simulink model "Control_Telegram"  (R2020b)
settings: Solver=FixedStepDiscrete  StartTime=0.0  StopTime=inf  FixedStep=0.01  RelTol=1e-3  EnableMultiTasking=on
libraries: arduinolib x12, simulink x4, pid_lib x2, commutil2 x1
settings Model: SILPILModeSetting=veronly  ExtModeTrigDuration=2  Creator=Lenovo  LastModifiedBy=Lenovo
settings SolverCC: AutoInsertRateTranBlk=on
settings OptimizationCC: EnhancedBackFolding=on  PassReuseOutputArgsAs=Individual arguments  ZeroExternalMemoryAtStartup=off  ZeroInternalMemoryAtStartup=off  MaxStackSize=64  OptimizeBlockOrder=speed  DifferentSizesBufferReuse=on  OptimizationCustomize=off  EfficientTunableParamExpr=on
settings DebuggingCC: MultiTaskDSMMsg=none  ParameterTunabilityLossMsg=error
settings HardwareCC: ProdBitPerInt=16  ProdBitPerPointer=16  ProdBitPerSizeT=16  ProdBitPerPtrDiffT=16  ProdLargestAtomicFloat=None  ProdWordSize=8  ProdHWDeviceType=Atmel->AVR
settings SFSimCC: MATLABDynamicMemAlloc=off
settings RTWCC: Description=Embedded Coder  SystemTargetFile=ert.tlc  HardwareBoard=Arduino Mega 2560  TemplateMakefile=ert_default_tmf  Toolchain=Arduino AVR  BuildConfiguration=Faster Runs
settings CodeAppCC: ForceParamTrailComments=on  IgnoreCustomStorageClasses=off  OperatorAnnotations=on  SimulinkDataObjDesc=on  SFDataObjDesc=on  InsertBlockDesc=on
settings ERTTargetCC: SupportContinuousTime=on  SupportVariableSizeSignals=on  ExtModeStaticAllocSize=2048

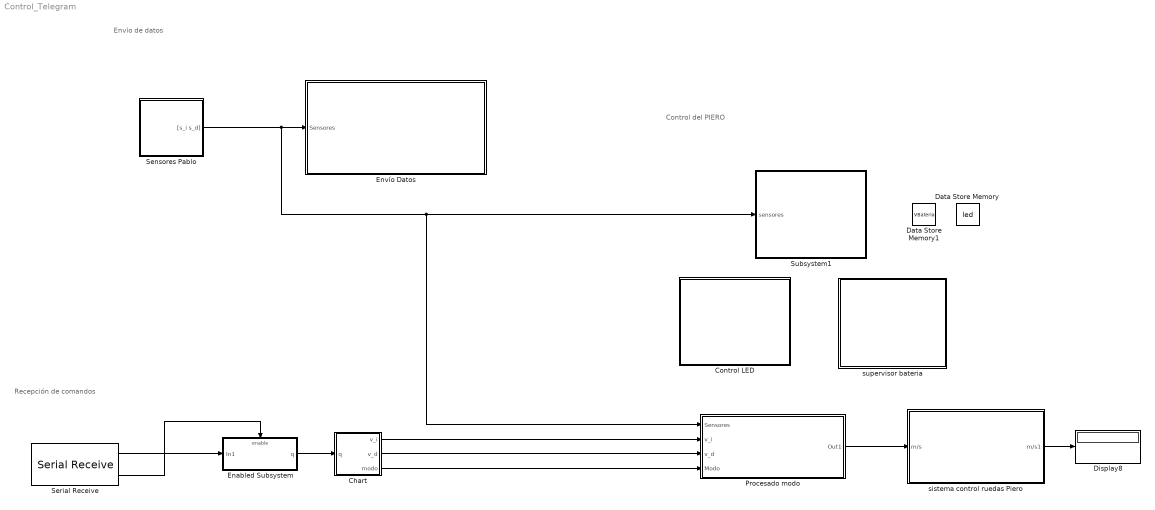
== system Control_Telegram ==
  note: Recepción de comandos
  note: Control del PIERO
  note: Envío de datos
  Chart : Stateflow chart  TreatAsAtomicUnit=on
      settings: PortSchema="{\"entries\":[{\"content\":{\"sides\":[{\"content\":{\"connectorIds\":[\"In1\"]},\"type\":\"ConnectorPlacement.EquallySpacedRectSide\",\"uuid\":\"460ffd16-b0a8-46f0-b413-d255944a2202\"},{\"content\":{\"connectorIds\":[\"Out2\",\"Out1\",\"Out3\"],\"side\":\"RIGHT\"},\"type\":\"ConnectorPlacement.EquallySpacedRectSide\",\"uuid\":\"2f6da82c-ccd3-4a6a-9034-5a862735bd5f\"},{\"content\":{\"connectorIds\":[],\"side\":\"TOP\"},\"type\":\"ConnectorPlacement.EquallySpacedRectSide\",\"uuid\":\"193d4201-0e4c-4dc7-8b4f-a6b3a7c4f850\"},{\"content\":{\"connectorIds\":[],\"side\":\"HIDDEN\"},\"type\":\"ConnectorPlacement.EquallySpacedRectSide\",\"uuid\":\"5c8087d8-0ec6-4d7b-ac7b-a5b39b248132\"}]},\"type\":\"ConnectorPlacement.EquallySpacedConnector\",\"uuid\":\"9f9eacda-d61e-4b8a-833c-1ceadcf75f15\"}],\"packageUris\":[\"http://schema.mathworks.com/mf0/Connector/R2020b\"],\"version\":\"1.0\"}"
  Control LED : Subsystem
      mask Display: image('C:\Users\Lenovo\Desktop\4ºGIERM\LAB ROB\RBG-LED.jpg'); % Use "Edit Image" on toolstrip to change.
  Data Store Memory : DataStoreMemory  DataStoreName=led  ReadBeforeWriteMsg=warning  WriteAfterWriteMsg=warning  WriteAfterReadMsg=warning  ShowAdditionalParam=off
  Data Store Memory1 : DataStoreMemory  DataStoreName=VBateria  ReadBeforeWriteMsg=warning  WriteAfterWriteMsg=warning  WriteAfterReadMsg=warning  ShowAdditionalParam=off
  Display8 : Display
  Enabled Subsystem : Subsystem  TreatAsAtomicUnit=on
  Envío Datos : Subsystem
  Procesado modo : Subsystem
  Sensores Pablo : Subsystem
      mask Display: image('C:\Users\Lenovo\Desktop\4ºGIERM\LAB ROB\sensor.jpg'); % Use "Edit Image" on toolstrip to change.
  Serial Receive : arduinolib/Serial Receive  isARMArch=off  portNumber=3  DataType=uint8  Datalength=1  SampleTime=0.01  showOutStatus=on  blockPlatform=arduino
      settings: SourceProductBaseCode=ARDUINO
  Subsystem1 : Subsystem
  sistema control ruedas Piero : Subsystem
  supervisor bateria : Subsystem
      mask Display: image('C:\Users\Lenovo\Desktop\4ºGIERM\LAB ROB\bateria.jpg'); % Use "Edit Image" on toolstrip to change.
  wires:
  Serial Receive/2 -> Enabled Subsystem/Enable
  Sensores Pablo/1("[s_i s_d]") -> Procesado modo/1(Sensores), Subsystem1/1(sensores), Envío Datos/1(Sensores)
  Enabled Subsystem/1(q) -> Chart/1(q)
  Serial Receive/1 -> Enabled Subsystem/1(In1)
  sistema control ruedas Piero/1(m/s1) -> Display8/1
  Chart/2(v_i) -> Procesado modo/2(v_i)
  Chart/1(v_d) -> Procesado modo/3(v_d)
  Chart/3(modo) -> Procesado modo/4(Modo)
  Procesado modo/1(Out1) -> sistema control ruedas Piero/1(m/s)

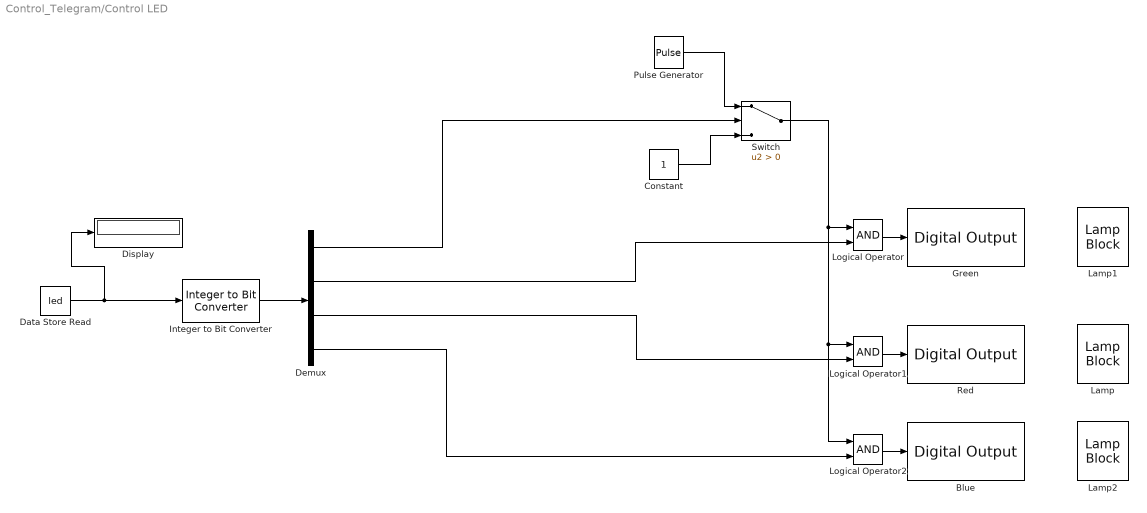
== system Control_Telegram/Control LED ==
  Blue : arduinolib/Digital Output  pinNumber=49  Direction=output  blockPlatform=arduino
  Constant : Constant
  Data Store Read : DataStoreRead  DataStoreName=led
  Demux : Demux
  Display : Display
  Green : arduinolib/Digital Output  pinNumber=53  Direction=output  blockPlatform=arduino
  Integer to Bit Converter : commutil2/Integer to Bit Converter  nbits=4  signedInputValues=Unsigned  bitOrder=MSB first  outDtype=Inherit via internal rule
  Lamp : LampBlock
  Lamp1 : LampBlock
  Lamp2 : LampBlock
  Logical Operator : Logic  AllPortsSameDT=off  OutDataTypeStr=boolean
  Logical Operator1 : Logic  AllPortsSameDT=off  OutDataTypeStr=boolean
  Logical Operator2 : Logic  AllPortsSameDT=off  OutDataTypeStr=boolean
  Pulse Generator : DiscretePulseGenerator  PulseType=Time based  Period=0.5  PulseWidth=50
  Red : arduinolib/Digital Output  pinNumber=51  Direction=output  blockPlatform=arduino
  Switch : Switch  Criteria=u2 > Threshold
  wires:
  Logical Operator/1 -> Green/1
  Logical Operator2/1 -> Blue/1
  Logical Operator1/1 -> Red/1
  Switch/1 -> Logical Operator2/1, Logical Operator1/1, Logical Operator/1
  Demux/1 -> Switch/2
  Pulse Generator/1 -> Switch/1
  Constant/1 -> Switch/3
  Data Store Read/1 -> Display/1, Integer to Bit Converter/1
  Demux/2 -> Logical Operator/2
  Demux/4 -> Logical Operator2/2
  Demux/3 -> Logical Operator1/2
  Integer to Bit Converter/1 -> Demux/1

== system Control_Telegram/Enabled Subsystem ==
  In1 : Inport
  Enable : EnablePort
  q : Outport
  wires:
  In1/1 -> q/1

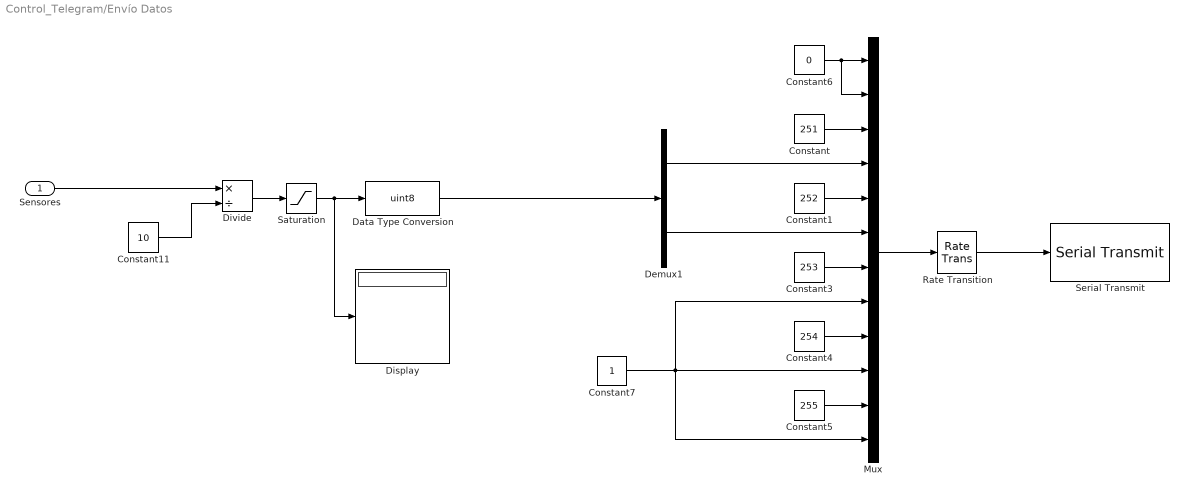
== system Control_Telegram/Envío Datos ==
  Sensores : Inport
  Constant : Constant  Value=251  OutDataTypeStr=uint8
  Constant1 : Constant  Value=252  OutDataTypeStr=uint8
  Constant11 : Constant  Value=10
  Constant3 : Constant  Value=253  OutDataTypeStr=uint8
  Constant4 : Constant  Value=254  OutDataTypeStr=uint8
  Constant5 : Constant  Value=255  OutDataTypeStr=uint8
  Constant6 : Constant  Value=0  OutDataTypeStr=uint8
  Constant7 : Constant  OutDataTypeStr=uint8
  Data Type Conversion : DataTypeConversion  OutMax=250  OutDataTypeStr=uint8
  Demux1 : Demux  Outputs=2
  Display : Display
  Divide : Product  Inputs=*/
  Mux : Mux  Inputs=12
  Rate Transition : RateTransition  OutPortSampleTime=0.9
  Saturation : Saturate  UpperLimit=255  LowerLimit=0
  Serial Transmit : arduinolib/Serial Transmit  portNumber=3  sendmode=write  label=sensores  sendformat=Decimal  floatprecision=2  blockPlatform=arduino
  wires:
  Constant5/1 -> Mux/11
  Rate Transition/1 -> Serial Transmit/1
  Constant3/1 -> Mux/7
  Constant6/1 -> Mux/2, Mux/1
  Saturation/1 -> Display/1, Data Type Conversion/1
  Demux1/1 -> Mux/4
  Constant4/1 -> Mux/9
  Mux/1 -> Rate Transition/1
  Constant1/1 -> Mux/5
  Divide/1 -> Saturation/1
  Data Type Conversion/1 -> Demux1/1
  Constant7/1 -> Mux/12, Mux/10, Mux/8
  Demux1/2 -> Mux/6
  Constant11/1 -> Divide/2
  Constant/1 -> Mux/3
  Sensores/1 -> Divide/1

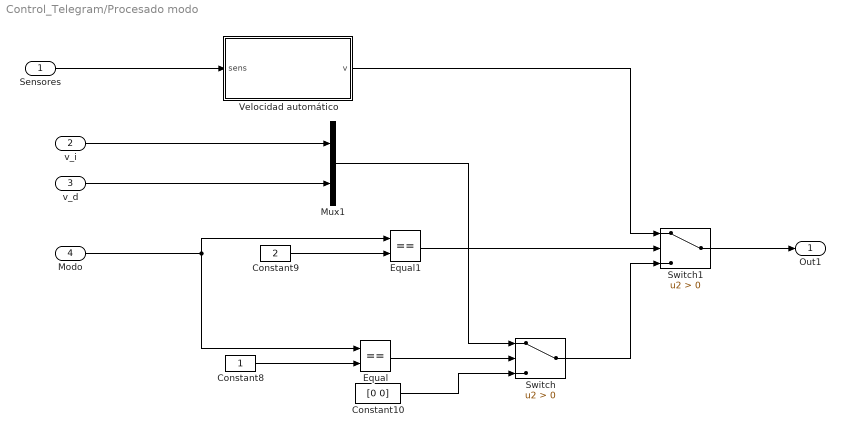
== system Control_Telegram/Procesado modo ==
  Sensores : Inport
  v_i : Inport  Port=2
  v_d : Inport  Port=3
  Modo : Inport  Port=4
  Constant10 : Constant  Value=[0 0]
  Constant8 : Constant
  Constant9 : Constant  Value=2
  Equal : RelationalOperator  Operator===  OutDataTypeStr=boolean  RndMeth=Simplest
  Equal1 : RelationalOperator  Operator===  OutDataTypeStr=boolean  RndMeth=Simplest
  Mux1 : Mux  Inputs=2
  Switch : Switch  Criteria=u2 > Threshold
  Switch1 : Switch  Criteria=u2 > Threshold
  Velocidad automático : Subsystem
  Out1 : Outport
  wires:
  Equal1/1 -> Switch1/2
  Equal/1 -> Switch/2
  Modo/1 -> Equal1/1, Equal/1
  Mux1/1 -> Switch/1
  Switch/1 -> Switch1/3
  v_d/1 -> Mux1/2
  Switch1/1 -> Out1/1
  Constant8/1 -> Equal/2
  Constant10/1 -> Switch/3
  Constant9/1 -> Equal1/2
  v_i/1 -> Mux1/1
  Sensores/1 -> Velocidad automático/1(sens)
  Velocidad automático/1(v) -> Switch1/1

== system Control_Telegram/Sensores Pablo ==
  Display2 : Display
  Display3 : Display
  Mux : Mux  Inputs=2
  SENSORES : Subsystem
  "[s_i s_d]" : Outport
  wires:
  SENSORES/2(Sensor Derecho) -> Mux/2, Display3/1
  SENSORES/1(Sensor Izquierdo) -> Mux/1, Display2/1
  Mux/1 -> "[s_i s_d]"/1

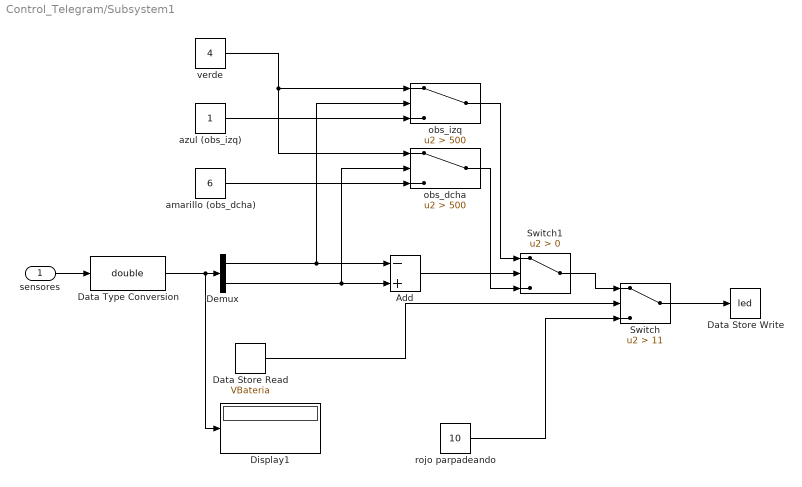
== system Control_Telegram/Subsystem1 ==
  sensores : Inport
  Add : Sum  Inputs=-+
  Data Store Read : DataStoreRead  DataStoreName=VBateria
  Data Store Write : DataStoreWrite  DataStoreName=led
  Data Type Conversion : DataTypeConversion  OutDataTypeStr=double
  Demux : Demux  Outputs=2
  Display1 : Display
  Switch : Switch  Criteria=u2 > Threshold  Threshold=11
  Switch1 : Switch  Criteria=u2 > Threshold
  amarillo (obs_dcha) : Constant  Value=6
  azul (obs_izq) : Constant
  obs_dcha : Switch  Criteria=u2 > Threshold  Threshold=500
  obs_izq : Switch  Criteria=u2 > Threshold  Threshold=500
  rojo parpadeando : Constant  Value=10
  verde : Constant  Value=4
  wires:
  Switch/1 -> Data Store Write/1
  rojo parpadeando/1 -> Switch/3
  sensores/1 -> Data Type Conversion/1
  verde/1 -> obs_izq/1, obs_dcha/1
  Demux/1 -> Add/1, obs_izq/2
  Demux/2 -> Add/2, obs_dcha/2
  azul (obs_izq)/1 -> obs_izq/3
  amarillo (obs_dcha)/1 -> obs_dcha/3
  Switch1/1 -> Switch/1
  Add/1 -> Switch1/2
  obs_izq/1 -> Switch1/1
  obs_dcha/1 -> Switch1/3
  Data Store Read/1 -> Switch/2
  Data Type Conversion/1 -> Display1/1, Demux/1

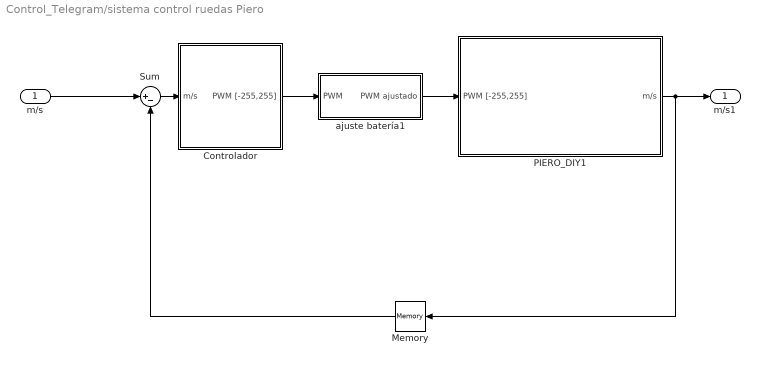
== system Control_Telegram/sistema control ruedas Piero ==
  m/s : Inport
  Controlador : Subsystem
  Memory : Memory
  PIERO_DIY1 : Subsystem
  Sum : Sum  Inputs=|+-
  ajuste batería1 : Subsystem
  m/s1 : Outport  VectorParamsAs1DForOutWhenUnconnected=off
  wires:
  Sum/1 -> Controlador/1(m/s)
  m/s/1 -> Sum/1
  PIERO_DIY1/1(m/s) -> Memory/1, m/s1/1
  Memory/1 -> Sum/2
  Controlador/1(PWM [-255,255]) -> ajuste batería1/1(PWM)
  ajuste batería1/1(PWM ajustado) -> PIERO_DIY1/1(PWM [-255,255])

== system Control_Telegram/supervisor bateria ==
  Bateria : arduinolib/Analog Input  pinNumber=0  ReadResultsOnly=off  ConversionTriggerSource=Software  ExternalTriggerType=uint32( 0 )  OutputDataType=uint16  EnableConversionCompleteNotify=off  EnableOuputStatus=off  SampleTime=1  blockPlatform=arduino
  Data Store Write1 : DataStoreWrite  DataStoreName=VBateria
  Gain : Gain  Gain=25/1023  OutDataTypeStr=double
  Quarter Gauge : QuarterGaugeBlock  ScaleMin=10  ScaleMax=13
  wires:
  Bateria/1 -> Gain/1
  Gain/1 -> Data Store Write1/1

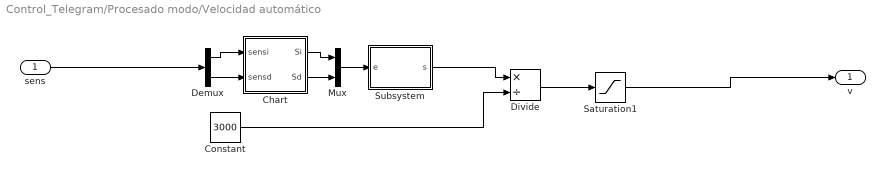
== system Control_Telegram/Procesado modo/Velocidad automático ==
  sens : Inport
  Chart : Stateflow chart  TreatAsAtomicUnit=on
  Constant : Constant  Value=3000
  Demux : Demux  Outputs=2
  Divide : Product  Inputs=*/
  Mux : Mux  Inputs=2
  Saturation1 : Saturate  UpperLimit=0.3  LowerLimit=0
  Subsystem : Subsystem
      settings: PortSchema="{\"entries\":[{\"content\":{\"sides\":[{\"content\":{\"connectorIds\":[]},\"type\":\"ConnectorPlacement.EquallySpacedRectSide\",\"uuid\":\"0a24279a-7a52-457c-98aa-c7ba1e82fcaa\"},{\"content\":{\"connectorIds\":[],\"side\":\"RIGHT\"},\"type\":\"ConnectorPlacement.EquallySpacedRectSide\",\"uuid\":\"0f762eb3-cf5d-4914-a9fc-c3582c9f6173\"},{\"content\":{\"connectorIds\":[\"In1\"],\"side\":\"TOP\"},\"type\":\"ConnectorPlacement.EquallySpacedRectSide\",\"uuid\":\"ea3e191d-7b8c-4d85-afaf-b1ec388f1efb\"},{\"content\":{\"connectorIds\":[\"Out1\"],\"side\":\"BOTTOM\"},\"type\":\"ConnectorPlacement.EquallySpacedRectSide\",\"uuid\":\"8d5bc53a-83b0-4fc8-aeef-cd0991329a34\"},{\"content\":{\"connectorIds\":[],\"side\":\"HIDDEN\"},\"type\":\"ConnectorPlacement.EquallySpacedRectSide\",\"uuid\":\"6d880959-49a3-460c-8ffc-802dbf3ca6c3\"}]},\"type\":\"ConnectorPlacement.EquallySpacedConnector\",\"uuid\":\"f1470ebd-e65e-4dba-8453-0009f24bd770\"}],\"packageUris\":[\"http://schema.mathworks.com/mf0/Connector/R2020b\"],\"version\":\"1.0\"}"
  v : Outport
  wires:
  Divide/1 -> Saturation1/1
  Saturation1/1 -> v/1
  Constant/1 -> Divide/2
  sens/1 -> Demux/1
  Demux/1 -> Chart/1(sensi)
  Chart/1(Si) -> Mux/1
  Demux/2 -> Chart/2(sensd)
  Chart/2(Sd) -> Mux/2
  Mux/1 -> Subsystem/1(e)
  Subsystem/1(s) -> Divide/1

== system Control_Telegram/Sensores Pablo/SENSORES ==
  Display : Display
  Display1 : Display
  S-Function Builder : S-Function  InitFcn=try, set_param(gcb,'FunctionName','Sensores_VL53L0X_I2C'), end  FunctionName=Sensores_VL53L0X_I2C  SFunctionModules=Sensores_VL53L0X_I2C_wrapper  SFunctionDeploymentMode=off  EnableBusSupport=off  mask(S-Function Builder){}
      mask help: Simulink:masks:SFunctionBuilder_MD
      mask init:
      | val = [[.9  0.75 0.75 1 1 .9 .9 1]',[1 1 0.75 0.75 .9 .9 1 .9]'];try , sys = get_param(gcb,'SfunBuilderFcnName');if isempty(sys), sys = get_param(gcb,'FunctionName'); end,catch, sys = get_param(gcb,'FunctionName'); end
      settings: CopyFcn=set_param(gcbh,'LinkStatus','none')  PreSaveFcn=try, set_param(gcb,'FunctionName','Sensores_VL53L0X_I2C'), end  OpenFcn=sfunctionwizard(gcbh)
      mask Display: plot(val(:,1),val(:,2)),disp(sys),port_label('output',1,'Sensor1'),port_label('output',2,'Sensor2')
  Sensor Izquierdo : Outport  VectorParamsAs1DForOutWhenUnconnected=off
  Sensor Derecho : Outport  Port=2  VectorParamsAs1DForOutWhenUnconnected=off
  wires:
  S-Function Builder/2 -> Display/1, Sensor Derecho/1
  S-Function Builder/1 -> Display1/1, Sensor Izquierdo/1

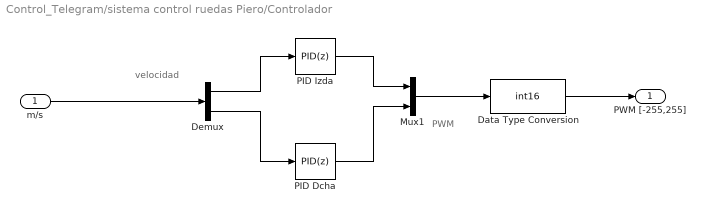
== system Control_Telegram/sistema control ruedas Piero/Controlador ==
  note: velocidad
  note: PWM
  m/s : Inport
  Data Type Conversion : DataTypeConversion  OutDataTypeStr=int16
  Demux : Demux  Outputs=2
  Mux1 : Mux  Inputs=2
  PID Dcha : pid_lib/PID Controller  Controller=PID  Form=Parallel  TimeDomain=Discrete-time  UseExternalTs=off  SampleTime=-1  IntegratorMethod=Forward Euler  FilterMethod=Forward Euler  ControllerParametersSource=internal  P=4.07505423535344  I=815.010847070688  D=0  UseFilter=on  N=100  TunerSelectOption=Transfer Function Based (PID Tuner App)  InitialConditionSource=internal  InitialConditionForIntegrator=0  InitialConditionForFilter=0  DifferentiatorICPrevScaledInput=0  ExternalReset=none  TrackingMode=off  Kt=1  LimitOutput=on  SatLimitsSource=internal  UpperSaturationLimit=255  LowerSaturationLimit=-255  LinearizeAsGain=on  AntiWindupMode=none  Kb=1  POutMin=[]  POutMax=[]  IOutMin=[]  IOutMax=[]  DOutMin=[]  DOutMax=[]  NOutMin=[]  NOutMax=[]  SumOutMin=[]  SumOutMax=[]  SaturationOutMin=[]  SaturationOutMax=[]  PParamMin=[]  PParamMax=[]  IParamMin=[]  IParamMax=[]  DParamMin=[]  DParamMax=[]  NParamMin=[]  NParamMax=[]  KbParamMin=[]  KbParamMax=[]  KtParamMin=[]  KtParamMax=[]  KbOutMin=[]  KbOutMax=[]  KtOutMin=[]  KtOutMax=[]  IntegratorOutMin=[]  IntegratorOutMax=[]  FilterOutMin=[]  FilterOutMax=[]  SumI1OutMin=[]  SumI1OutMax=[]  SumI2OutMin=[]  SumI2OutMax=[]  SumI3OutMin=[]  SumI3OutMax=[]  SumI4OutMin=[]  SumI4OutMax=[]  SumDOutMin=[]  SumDOutMax=[]  DifferentiatorOutMin=[]  DifferentiatorOutMax=[]  FilterDiffOutCoefMin=[]  FilterDiffOutCoefMax=[]  ReciprocalOutMin=[]  ReciprocalOutMax=[]  SumDenOutMin=[]  SumDenOutMax=[]  SumNumOutMin=[]  SumNumOutMax=[]  DivideOutMin=[]  DivideOutMax=[]  UdiffTsProdOutMin=[]  UdiffTsProdOutMax=[]  NTsProdOutMin=[]  NTsProdOutMax=[]  UintegralTsProdOutMin=[]  UintegralTsProdOutMax=[]  UngainTsProdOutMin=[]  UngainTsProdOutMax=[]  IntegratorContinuousStateAttributes=''  IntegratorStateMustResolveToSignalObject=off  IntegratorRTWStateStorageClass=Auto  FilterContinuousStateAttributes=''  FilterStateMustResolveToSignalObject=off  FilterRTWStateStorageClass=Auto  ParallelPVariant=InternalParameters  IdealPVariant=Disabled  IVariant=InternalParameters  DVariant=InternalParameters  IntegratorVariant=Discrete  SatVariant=Enabled  AWVariant=Passthrough  PCopyVariant=Disabled  TRVariant=Disabled  FdbkBlocksVariant=Forward  IdealPFdbkVariant=Disabled  SatFdbkVariant=Disabled  DerivativeFilterVariant=ForwardEulerFilter  NVariant=InternalParameters  NCopyVariant=Disabled  FilterICVariant=InternalICsFilter  IntegratorICVariant=InternalICs  ExternalResetVariant=Disabled  TRSumVariant=Passthrough  SumFdbkVariant=Disabled  SumVariant=Sum_PID  TsampFilterVariant=InternalTs  TsampNgainVariant=Passthrough  TsampIntegralVariant=Passthrough  ExternalSaturationOutDataTypeStr=Inherit: Same as second input
  PID Izda : pid_lib/PID Controller  Controller=PID  Form=Parallel  TimeDomain=Discrete-time  UseExternalTs=off  SampleTime=-1  IntegratorMethod=Forward Euler  FilterMethod=Forward Euler  ControllerParametersSource=internal  P=4.09864222198202  I=819.728444396404  D=0  UseFilter=on  N=100  TunerSelectOption=Transfer Function Based (PID Tuner App)  InitialConditionSource=internal  InitialConditionForIntegrator=0  InitialConditionForFilter=0  DifferentiatorICPrevScaledInput=0  ExternalReset=none  TrackingMode=off  Kt=1  LimitOutput=on  SatLimitsSource=internal  UpperSaturationLimit=255  LowerSaturationLimit=-255  LinearizeAsGain=on  AntiWindupMode=none  Kb=1  POutMin=[]  POutMax=[]  IOutMin=[]  IOutMax=[]  DOutMin=[]  DOutMax=[]  NOutMin=[]  NOutMax=[]  SumOutMin=[]  SumOutMax=[]  SaturationOutMin=[]  SaturationOutMax=[]  PParamMin=[]  PParamMax=[]  IParamMin=[]  IParamMax=[]  DParamMin=[]  DParamMax=[]  NParamMin=[]  NParamMax=[]  KbParamMin=[]  KbParamMax=[]  KtParamMin=[]  KtParamMax=[]  KbOutMin=[]  KbOutMax=[]  KtOutMin=[]  KtOutMax=[]  IntegratorOutMin=[]  IntegratorOutMax=[]  FilterOutMin=[]  FilterOutMax=[]  SumI1OutMin=[]  SumI1OutMax=[]  SumI2OutMin=[]  SumI2OutMax=[]  SumI3OutMin=[]  SumI3OutMax=[]  SumI4OutMin=[]  SumI4OutMax=[]  SumDOutMin=[]  SumDOutMax=[]  DifferentiatorOutMin=[]  DifferentiatorOutMax=[]  FilterDiffOutCoefMin=[]  FilterDiffOutCoefMax=[]  ReciprocalOutMin=[]  ReciprocalOutMax=[]  SumDenOutMin=[]  SumDenOutMax=[]  SumNumOutMin=[]  SumNumOutMax=[]  DivideOutMin=[]  DivideOutMax=[]  UdiffTsProdOutMin=[]  UdiffTsProdOutMax=[]  NTsProdOutMin=[]  NTsProdOutMax=[]  UintegralTsProdOutMin=[]  UintegralTsProdOutMax=[]  UngainTsProdOutMin=[]  UngainTsProdOutMax=[]  IntegratorContinuousStateAttributes=''  IntegratorStateMustResolveToSignalObject=off  IntegratorRTWStateStorageClass=Auto  FilterContinuousStateAttributes=''  FilterStateMustResolveToSignalObject=off  FilterRTWStateStorageClass=Auto  ParallelPVariant=InternalParameters  IdealPVariant=Disabled  IVariant=InternalParameters  DVariant=InternalParameters  IntegratorVariant=Discrete  SatVariant=Enabled  AWVariant=Passthrough  PCopyVariant=Disabled  TRVariant=Disabled  FdbkBlocksVariant=Forward  IdealPFdbkVariant=Disabled  SatFdbkVariant=Disabled  DerivativeFilterVariant=ForwardEulerFilter  NVariant=InternalParameters  NCopyVariant=Disabled  FilterICVariant=InternalICsFilter  IntegratorICVariant=InternalICs  ExternalResetVariant=Disabled  TRSumVariant=Passthrough  SumFdbkVariant=Disabled  SumVariant=Sum_PID  TsampFilterVariant=InternalTs  TsampNgainVariant=Passthrough  TsampIntegralVariant=Passthrough  ExternalSaturationOutDataTypeStr=Inherit: Same as second input
  PWM [-255,255] : Outport  VectorParamsAs1DForOutWhenUnconnected=off
  wires:
  PID Izda/1 -> Mux1/1
  Demux/1 -> PID Izda/1
  Demux/2 -> PID Dcha/1
  Mux1/1 -> Data Type Conversion/1
  PID Dcha/1 -> Mux1/2
  Data Type Conversion/1 -> PWM [-255,255]/1
  m/s/1 -> Demux/1

== system Control_Telegram/sistema control ruedas Piero/PIERO_DIY1 ==
  PWM [-255,255] : Inport
  Environment Controller : simulink/Signal Routing/Environment Controller
      settings: SourceProductBaseCode=SL
  Modelo PieroDIY : Subsystem
  PieroDIY-HW : Subsystem
  m/s : Outport  VectorParamsAs1DForOutWhenUnconnected=off
  wires:
  PWM [-255,255]/1 -> Modelo PieroDIY/1(PWM -255,255), PieroDIY-HW/1(PWM 255_-255)
  Environment Controller/1 -> m/s/1
  PieroDIY-HW/1(metros/segundo) -> Environment Controller/2
  Modelo PieroDIY/1(m/s) -> Environment Controller/1

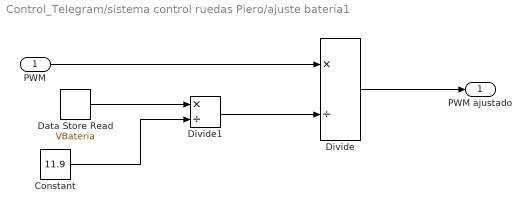
== system Control_Telegram/sistema control ruedas Piero/ajuste batería1 ==
  PWM : Inport
  Constant : Constant  Value=11.9
  Data Store Read : DataStoreRead  DataStoreName=VBateria
  Divide : Product  Inputs=*/
  Divide1 : Product  Inputs=*/
  PWM ajustado : Outport
  wires:
  PWM/1 -> Divide/1
  Divide/1 -> PWM ajustado/1
  Divide1/1 -> Divide/2
  Data Store Read/1 -> Divide1/1
  Constant/1 -> Divide1/2

== system Control_Telegram/Procesado modo/Velocidad automático/Subsystem ==
  e : Inport
  Demux2 : Demux  Outputs=2
  Mux2 : Mux  Inputs=2
  s : Outport
  wires:
  Demux2/1 -> Mux2/2
  Demux2/2 -> Mux2/1
  e/1 -> Demux2/1
  Mux2/1 -> s/1

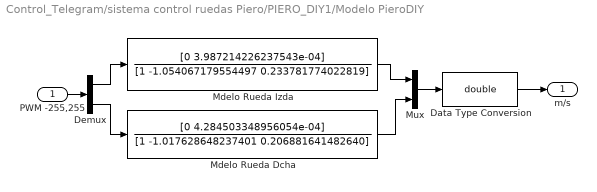
== system Control_Telegram/sistema control ruedas Piero/PIERO_DIY1/Modelo PieroDIY ==
  PWM -255,255 : Inport
  Data Type Conversion : DataTypeConversion  OutDataTypeStr=double
  Demux : Demux  Outputs=2
  Mdelo Rueda Dcha : DiscreteFilter  Numerator=[0 4.284503348956054e-04]  Denominator=[1 -1.017628648237401 0.206881641482640]
  Mdelo Rueda Izda : DiscreteFilter  Numerator=[0 3.987214226237543e-04]  Denominator=[1 -1.054067179554497 0.233781774022819]
  Mux : Mux  Inputs=2
  m/s : Outport  VectorParamsAs1DForOutWhenUnconnected=off
  wires:
  Demux/2 -> Mdelo Rueda Dcha/1
  Demux/1 -> Mdelo Rueda Izda/1
  Mdelo Rueda Izda/1 -> Mux/1
  Mdelo Rueda Dcha/1 -> Mux/2
  Mux/1 -> Data Type Conversion/1
  PWM -255,255/1 -> Demux/1
  Data Type Conversion/1 -> m/s/1

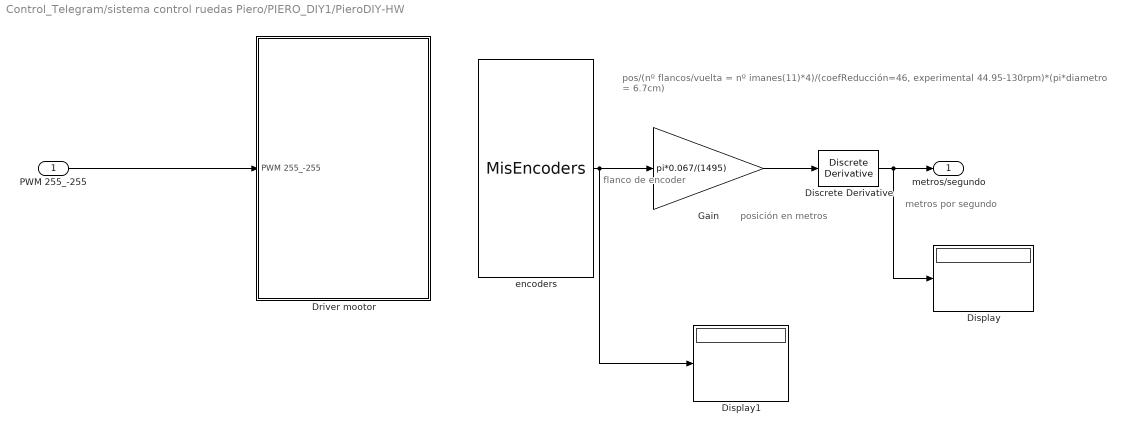
== system Control_Telegram/sistema control ruedas Piero/PIERO_DIY1/PieroDIY-HW ==
  note: metros por segundo
  note: posición en metros
  note: pos/(nº flancos/vuelta = nº imanes(11)*4)/(coefReducción=46, experimental 44.95-130rpm)*(pi*diametro = 6.7cm)
  note: flanco de encoder
  PWM 255_-255 : Inport
  Discrete Derivative : simulink/Discrete/Discrete Derivative  gainval=1.0  ICPrevScaledInput=0.0  OutMin=[]  OutMax=[]  OutDataTypeStr=double  OutputDataTypeScalingMode=double  OutDataType=fixdt(1, 16)  OutScaling=2^-10  DoSatur=off
  Display : Display
  Display1 : Display
  Driver mootor : Subsystem
  Gain : Gain  Gain=pi*0.067/(1495)
  encoders : S-Function  InitFcn=try, set_param(gcb,'FunctionName','MisEncoders'), end  FunctionName=MisEncoders  Parameters=uint8(0),uint8(2),uint8(3),uint8(1),uint8(19),uint8(18)  SFunctionModules=MisEncoders_wrapper  SFunctionDeploymentMode=off  EnableBusSupport=off  mask(S-Function Builder){}
      mask help: Simulink:masks:SFunctionBuilder_MD
      mask init: same as Control_Telegram/Sensores Pablo/SENSORES/S-Function Builder
      settings: CopyFcn=set_param(gcbh,'LinkStatus','none')  PreSaveFcn=try, set_param(gcb,'FunctionName','MisEncoders'), end  OpenFcn=sfunctionwizard(gcbh)
      mask Display: plot(val(:,1),val(:,2)),disp(sys),port_label('output',1,'pos')
  metros/segundo : Outport  VectorParamsAs1DForOutWhenUnconnected=off
  wires:
  PWM 255_-255/1 -> Driver mootor/1(PWM 255_-255)
  encoders/1 -> Gain/1, Display1/1
  Discrete Derivative/1 -> Display/1, metros/segundo/1
  Gain/1 -> Discrete Derivative/1

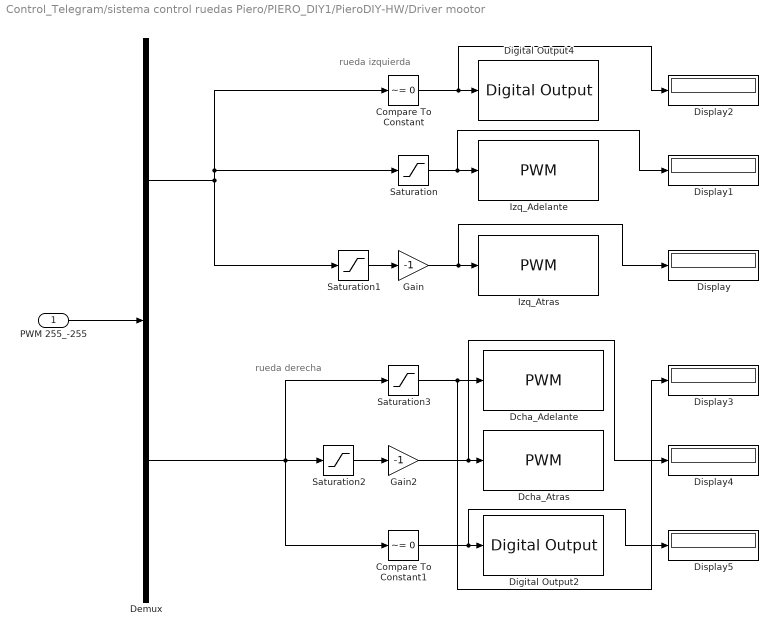
== system Control_Telegram/sistema control ruedas Piero/PIERO_DIY1/PieroDIY-HW/Driver mootor ==
  note: rueda derecha
  note: rueda izquierda
  PWM 255_-255 : Inport
  Compare To Constant : simulink/Logic and Bit Operations/Compare To Constant  relop=~=  const=0  OutDataTypeStr=boolean
  Compare To Constant1 : simulink/Logic and Bit Operations/Compare To Constant  relop=~=  const=0  OutDataTypeStr=boolean
  Dcha_Adelante : arduinolib/PWM  pinNumber=8  frequencyType=Default  desiredFrequency=490.2  achievableFrequency=490.2
  Dcha_Atras : arduinolib/PWM  pinNumber=7  frequencyType=Default  desiredFrequency=490.2  achievableFrequency=490.2
  Demux : Demux  Outputs=2
  Digital Output2 : arduinolib/Digital Output  pinNumber=6  Direction=output  blockPlatform=arduino
  Digital Output4 : arduinolib/Digital Output  pinNumber=11  Direction=output  blockPlatform=arduino
  Display{,1..5} (6 alike) : Display
  Gain : Gain  Gain=-1  OutDataTypeStr=uint8
  Gain2 : Gain  Gain=-1  OutDataTypeStr=uint8
  Izq_Adelante : arduinolib/PWM  pinNumber=9  frequencyType=Default  desiredFrequency=490.2  achievableFrequency=490.2
  Izq_Atras : arduinolib/PWM  pinNumber=10  frequencyType=Default  desiredFrequency=490.2  achievableFrequency=490.2
  Saturation : Saturate  UpperLimit=255  LowerLimit=0
  Saturation1 : Saturate  UpperLimit=0  LowerLimit=-255
  Saturation2 : Saturate  UpperLimit=0  LowerLimit=-255
  Saturation3 : Saturate  UpperLimit=255  LowerLimit=0
  wires:
  Compare To Constant1/1 -> Display5/1, Digital Output2/1
  Saturation3/1 -> Dcha_Adelante/1, Display3/1
  Compare To Constant/1 -> Display2/1, Digital Output4/1
  Saturation2/1 -> Gain2/1
  Saturation/1 -> Display1/1, Izq_Adelante/1
  PWM 255_-255/1 -> Demux/1
  Demux/1 -> Saturation1/1, Saturation/1, Compare To Constant/1
  Saturation1/1 -> Gain/1
  Gain/1 -> Display/1, Izq_Atras/1
  Demux/2 -> Compare To Constant1/1, Saturation2/1, Saturation3/1
  Gain2/1 -> Display4/1, Dcha_Atras/1

== stateflow chart Control_Telegram/Procesado modo/Velocidad automático/Chart ==
  settings: updateMethod=DISCRETE  sampleTime=0.03
  state inicio
    Si=sensi;
    Sd=sensd;
  state izquierda_muy_cercano
    Si=0;
    Sd=sensd;
  state derecha_muy_cercano1
    Sd=0;
    Si=sensi;
  (default) -> inicio
  inicio -> izquierda_muy_cercano [order 1] : [sensi<250]
  inicio -> derecha_muy_cercano1 [order 2] : [sensd<250]
  izquierda_muy_cercano -> inicio : [sensi>250]
  derecha_muy_cercano1 -> inicio : [sensd>250]
  data: sensi input; sensd input; Si output; Sd output

== stateflow chart Control_Telegram/Chart ==
  state Modo2 Reposo [group]
    state nada
      v_i=0;
      v_d=0;
      modo=0;
    state espera1
    state Primera_etiqueta_X1
    (default) -> nada
    Primera_etiqueta_X1 -> nada [order 1] : [q=='R']
    nada -> espera1
    espera1 -> Primera_etiqueta_X1 : [q=='X']
  state Modo1 Automático [group]
    state Evita_obs
      entry:
      modo=2;
  state Modo Manual [group]
    state espera
      entry:
      modo=1;
    state Derecha
      entry:
      if(v_i<=0.35)
      v_i=v_i+0.05;
      end
      if (v_d>=-0.2)
      v_d=v_d-0.02;
      end;
    state Izquierda
      entry:
      if(v_d<=0.35)
      v_d=v_d+0.05;
      end
      if (v_i>=-0.2)
      v_i=v_i-0.02;
      end;
    state Primera_etiqueta_X
    state Adelante
      entry:
      if(v_i<=0.35 & v_d<=0.35)
      v_i=v_i+0.05;
      v_d=v_d+0.05;
      end;
    state Parar
      entry:
      v_i=0;
      v_d=0;
    state Atras
      entry:
      if(v_d>=-0.2 & v_i>=-0.2)
      v_d=v_d-0.05;
      v_i=v_i-0.05;
      end;
    Derecha -> espera
    Izquierda -> espera
    Atras -> espera
    Parar -> espera
    Adelante -> espera
    Primera_etiqueta_X -> espera [order 7] : [q=='M']
    espera -> Primera_etiqueta_X : [q=='X']
    Primera_etiqueta_X -> Izquierda [order 1] : [q=='A']
    Primera_etiqueta_X -> Derecha [order 3] : [q=='D']
    Primera_etiqueta_X -> Adelante [order 4] : [q=='W']
    Primera_etiqueta_X -> Parar [order 6] : [q==' ']
    Primera_etiqueta_X -> Atras [order 5] : [q=='S']
  Primera_etiqueta_X -> nada [order 2] : [q=='R']
  Evita_obs -> Primera_etiqueta_X1 : [q=='X']
  Primera_etiqueta_X1 -> Evita_obs [order 3] : [q=='E']
  Primera_etiqueta_X1 -> espera [order 2] : [q=='M']
  data: q input; v_d output; v_i output; modo output
